simulink model "DR18E_Testpult"  (R2017a)
settings: Solver=ode1  StartTime=0.0  StopTime=Inf  FixedStep=0.001  RelTol=1e-3
PostLoadFcn:
  | , if any(exist('dsrtsu_mdlpostloadfcn', 'file') == [2, 3, 6]), try dsrtsu_mdlpostloadfcn('Execute', bdroot); catch fprintf('Error in PostLoadFcn (dsrtsu_mdlpostloadfcn) for model "%s":\n %s\n', bdroot, lasterr); end, end,
model workspace: external: MATLAB File C:\Users\DeltaRacing\Documents\dSPACE\MABX_DR18E\Model\DR18E_MABX_Parameter.m (data not in the file)
values from neighbouring files (symbols this model uses):
  am = 1/Ts    (= 1)    [DR18E_MABX_Parameter.m]
  bm = K/Ts    (= 0.05)    [DR18E_MABX_Parameter.m]
  cf = 41350    [DR18E_MABX_Parameter.m]
  cr = 41350    [DR18E_MABX_Parameter.m]
  Derating_HV_Battery_Kapa = 1    [DR18E_MABX_Parameter.m]
  Derating_Start_km = 16    [DR18E_MABX_Parameter.m]
  Drive_Mode = 0    [DR18E_MABX_Parameter.m]
  g = 1    [DR18E_MABX_Parameter.m]
  Gas_Modus = 2    [DR18E_MABX_Parameter.m]
  HV_Power_max = 80    [DR18E_MABX_Parameter.m]
  i_Getriebe = 3.3    [DR18E_MABX_Parameter.m]
  i_Lenkgetriebe = 4.32    [DR18E_MABX_Parameter.m]
  K_SET = 1    [DR18E_MABX_Parameter.m]
  Kapazitaet_HV_Battery_kWh = 6.6    [DR18E_MABX_Parameter.m]
  KW_T_Soll = 37    [DR18E_MABX_Parameter.m]
  lf = 1.2    [DR18E_MABX_Parameter.m]
  lr = 1.15    [DR18E_MABX_Parameter.m]
  m = 310    [DR18E_MABX_Parameter.m]
  M_max = 150    [DR18E_MABX_Parameter.m]
  Power_Limit_onoff = 0    [DR18E_MABX_Parameter.m]
  Reifenradius = 0.2351    [DR18E_MABX_Parameter.m]
  Strecke_Endu_km = 22    [DR18E_MABX_Parameter.m]
  TC_Decr_Gas = 0.00005    (= 5e-05)    [DR18E_MABX_Parameter.m]
  TC_Derivative = 0.4    [DR18E_MABX_Parameter.m]
  TC_Incr_Gas = 0.005    [DR18E_MABX_Parameter.m]
  TC_On = 0    [DR18E_MABX_Parameter.m]
  TC_Relay_Off = 0.065    [DR18E_MABX_Parameter.m]
  TC_Relay_On = 0.07    [DR18E_MABX_Parameter.m]
  TV_Mode = 2    [DR18E_MABX_Parameter.m]
  TV_On = 0    [DR18E_MABX_Parameter.m]
  TV_Override = 1    [DR18E_MABX_Parameter.m]
  y = 0.8    [DR18E_MABX_Parameter.m]
undefined symbols (not defined in the file or in its folder): D, DiscIntNeverNeededParam, I, K_OL, P
libraries: simulink x288, rtican x105, rtiusbflightreclib x40, rti1401lib_dio_type3 x10, simulink_extras x10, rti1401lib_adc_type4 x8, rti1401lib_II_base x7
(part 16 of 28)

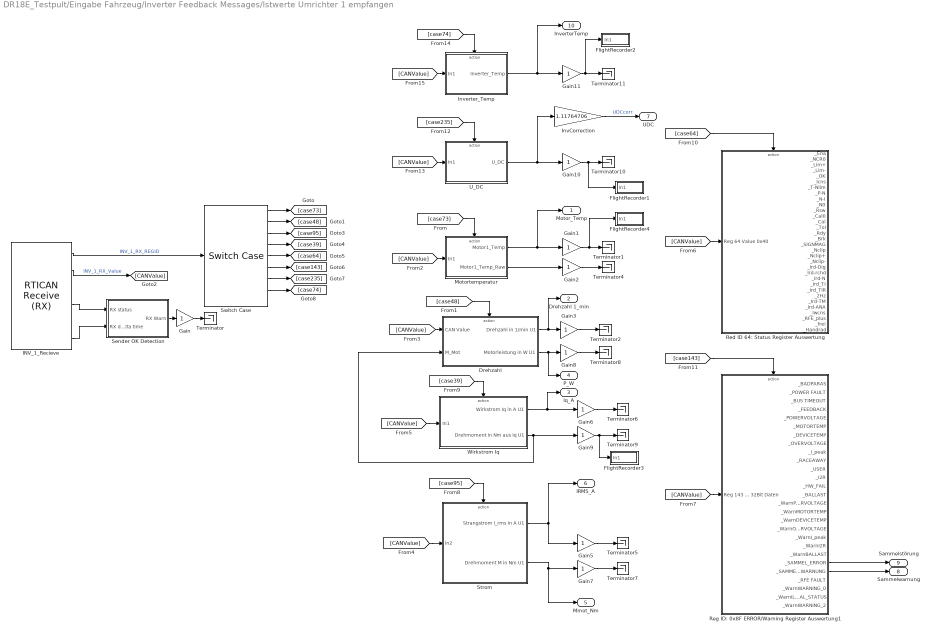
== system DR18E_Testpult/Eingabe Fahrzeug/Inverter Feedback Messages/Istwerte Umrichter 1 empfangen  ==
  Drehzahl : Subsystem  TreatAsAtomicUnit=on
  FlightRecorder1 : Subsystem
  FlightRecorder2 : Subsystem
  FlightRecorder3 : Subsystem
  FlightRecorder4 : Subsystem
  Gain{,1..3,5..11} (11 alike) : Gain
  INV_1_Recieve : rtican/RTICAN Receive (RX)   Reserved1=[]  Reserved2=[]  Reserved3=[]  Reserved4=[]  SfcnMessage=[]  Msg_Struct=[]  BoardTypeNo=[]  BoardNo=[]  ChannelNo=[]  Parameters=[]  DialogFcn=[]  UnitName=[]  Revision=[]  UnitValues=[]  DSProperties=struct('RTI',struct('Version',uint32(5),'BlockType',struct('isSLSource',uint8(1),'isSLSink',uint8(1),'isHWSource',uint8(0),'isHWSink',uint8(0),'isSetup',uint8(0),'isInline',uint8(1),'isNonInline',uint8(0),'isInterrupt',uint8(0),'isChannelwise',uint8(0)),'IOBoardType','RTICAN','UnitType','MESSAGE','Identifier','RX','DialogType','MSVC','BlockSet','RTICAN','SlaveProcessor','CAN'))  RTIBlockInterface=struct('OutputPortsWidth',int32([1 1 1 1 1 1]),'OutputPortsActive',[1 1 1 1 1 1],'OutputPortsName',{{'INV_1_RX_REGID','INV_1_RX_Value','muell',['RX status'],['RX time'],['RX delta time']}},'OutputPortsDataType',{{'SS_DOUBLE','SS_DOUBLE','SS_DOUBLE','SS_DOUBLE','SS_DOUBLE','SS_DOUBLE'}},'OutputPortsLabel',{{'INV_1_RX_REGID','INV_1_RX_Value','muell','','',''}},'OutputPortsLabelMode','ON','InputPortsWidth',int32(0),'InputPortsActive',0,'DialogFcn','rtican_message_interface_gui','BlockDisplay',{{'','center'}},'IconTransparency','on','ParameterTunableNames',{{}},'InitLevel',3,'BlockName',struct('Token',{{'INV_1_Recieve'}}),'SampleTime',{{-1}},'TriggerPort',{{'none'}},'EnablePort',{{'none'}})  RTIBlockParameters=struct('BoardTypeNo',{{1,'OFF',[]}},'BoardNo',{{1,'ON',[1 16]}},'ChannelNo',{{1,'ON',[1 2]}},'Parameters',{{struct('DataFileSupport',struct('DataFileSelectedMaster',0,'DataFileSelectedLocal',0,'DataFileName',['<no datafile support>|'],'DataFileDate',['01-Aug-2018 13:44:51'],'SelectedFile',['<no file selected>'],'InterfaceFcn','rtican_dbc_file_parser'),'Options',struct('StatusSelected',1,'TimeSelected',1,'DeltaTimeSelected',1,'BytePortSelected',0,'MessageLengthSelected',0,'TriggerPort',struct('Selected',0,'TriggerType',0),'UserCoding',struct('Selected',0,'InterfaceFile','UserDecodingFile','FcnName','UserDecodeFcn','InportSelected',0,'InportWidth',1,'OutportSelected',0,'OutportWidth',1),'EnablePortSelected',0,'SignalOnPortnameSelected',1,'UseRXService',0),'Message',struct('MsgOnBlocknameSelected',1,'MsgName','INV_1_Recieve','MsgIdFormat',0,'MsgId',273,'MsgLength',6,'NumSignals',3,'SampleTime',-1,'Signal',struct('SgnName',{'INV_1_RX_REGID','INV_1_RX_Value','muell'},'SgnStartBit',{0,8,40},'SgnLength',{8,16,8},'SgnType',{0,0,0},'ModeValue',{-1,-1,-1},'DataType',{0,0,0},'ByteLayout',{0,0,0},'Factor',{1,1,1},'Offset',{0,0,0},'SgnComment',{{''},{''},{''}},'SgnUnit',{'','',''},'Min',{0,0,0},'Max',{0,0,0},'SLDataType',{'SS_DOUBLE','SS_DOUBLE','SS_DOUBLE'}),'MsgIdNumFormat',1,'MsgComment',{{''}}),'Version',1.2,'general',struct('isFromLib',0)),'OFF',[]}},'GroupId',{{struct('Group',{{'RTICAN'}},'No',2,'Behavior',{{'NAMECHANGE'}},'BlockType',{{'SINK'}},'NameChangeFlag',0),'OFF',[]}},'SFcnRTICANMessage',{{struct('MsgType','RX','SFcnPortType','Scalar','MsgName','INV_1_Recieve','MsgIdFormat','STD','MsgId',273,'MsgLength',6,'NumSignals',3,'SampleTime',-1,'Signal',struct('SgnName',{'INV_1_RX_REGID','INV_1_RX_Value','muell'},'SgnStartBit',{0,8,40},'SgnLength',{8,16,8},'SgnType',{'standard','standard','standard'},'ModeValue',{-1,-1,-1},'DataType',{['unsigned int'],['unsigned int'],['unsigned int']},'ByteLayout',{['little endian'],['little endian'],['little endian']},'Factor',{1,1,1},'Offset',{0,0,0},'SLDataType',{'SS_DOUBLE','SS_DOUBLE','SS_DOUBLE'}),'StatusSelected','yes','TimeSelected','yes','DeltaTimeSelected','yes','BytePortSelected','no','MessageLengthSelected','no','TriggerPort',struct('Selected','no','TriggerType',0),'UserCoding',struct('Selected','no','InterfaceFile','UserDecodingFile','FcnName','UserDecodeFcn','InportSelected','no','InportWidth',1,'OutportSelected','no','OutportWidth',1),'EnablePortSelected','no','UseRXService','no','BoardType','DS1','BoardNo',1,'ControllerNo',1),'OFF',[]}},'TLCFileName',{{'rtican_rx_message','OFF',[]}})  RTISFcnParameters=struct('SFcnRTICANMessage','struct','TLCFileName','char')  RTIBlockParaDefault=struct('BoardTypeNo',4302,'BoardNo',1,'ChannelNo',1,'Parameters',struct('DataFileSupport',struct('DataFileSelectedMaster',0,'DataFileSelectedLocal',0,'DataFileName','','DataFileDate','','SelectedFile',['<no file selected>']),'Options',struct('StatusSelected',1,'TimeSelected',1,'DeltaTimeSelected',1,'BytePortSelected',0,'MessageLengthSelected',0,'TriggerPort',struct('Selected',0,'TriggerType','rising'),'UserCoding',struct('Selected',0,'InterfaceFile','UserDecodingFile','FcnName','UserDecodeFcn','InportSelected',0,'InportWidth',1,'OutportSelected',0,'OutportWidth',1),'EnablePortSelected',0,'SignalOnPortnameSelected',1,'UseRXService',0),'Message',struct('MsgOnBlocknameSelected',0,'MsgName',['RX Message'],'MsgIdFormat',0,'MsgId',100,'MsgLength',8,'NumSignals',1,'SampleTime',-1,'Signal',struct('SgnName',['RX signal'],'SgnStartBit',0,'SgnLength',8,'SgnType',0,'ModeValue',-1,'DataType',0,'SLDataType','SS_DOUBLE','ByteLayout',0,'Factor',1,'Offset',0,'Min',0,'Max',255,'SgnComment',{{}},'SgnUnit',''),'MsgIdNumFormat',0,'MsgComment',{{''}}),'Version',1.2,'general',struct('isFromLib',1)),'GroupId',struct('Group',{{'RTICAN'}},'No',1,'Behavior',{{'NAMECHANGE'}},'BlockType',{{'SINK'}},'NameChangeFlag',0),'SFcnRTICANMessage',struct('MsgType','RX','MsgName',['RX Message'],'MsgIdFormat','STD','MsgId',100,'MsgLength',8,'NumSignals',1,'SampleTime',-1,'Signal',struct('SgnName',['RX signal'],'SgnStartBit',0,'SgnLength',8,'SgnType','standard','ModeValue',-1,'DataType',['unsigned int'],'ByteLayout',['little endian'],'SLDataType','SS_DOUBLE','Factor',1,'Offset',0),'StatusSelected','yes','TimeSelected','yes','DeltaTimeSelected','yes','BytePortSelected','no','MessageLengthSelected','no','EnablePortSelected','no','UserCoding',struct('Selected','no','InterfaceFile','UserDecodingFile','FcnName','UserDecodeFcn','InportSelected','no','InportWidth',1,'OutportSelected','no','OutportWidth',1),'TriggerPort',struct('Selected','no','TriggerType','rising'),'UseRXService','no','BoardType','DS4302','BoardNo',1,'ControllerNo',1,'SFcnPortType','Scalar'),'TLCFileName','rtican_rx_message')
      settings: AttributesFormatString=Group Id: RTICAN2\n  SourceProductName=dSPACE RTI CAN Blockset
  InvCorrection : Gain  Gain=1.11764706
  Inverter_Temp : Subsystem  TreatAsAtomicUnit=on
  Motortemperatur : Subsystem  TreatAsAtomicUnit=on
  Red ID 64: Status Register Auswertung : Subsystem  TreatAsAtomicUnit=on
  Reg ID: 0x8F ERROR/Warning Register Auswertung1 : Subsystem  TreatAsAtomicUnit=on
  Sender OK Detection : Subsystem
  Strom : Subsystem  TreatAsAtomicUnit=on
  Switch Case : SwitchCase  CaseConditions={hex2dec('0049'),hex2dec('0030'),hex2dec('005F'),hex2dec('27'),64,hex2dec('8F'),hex2dec('EB'),hex2dec('4A')}
  Terminator{,1..2,4..11} (11 alike) : Terminator
  U_DC : Subsystem  TreatAsAtomicUnit=on
  Wirkstrom Iq : Subsystem  TreatAsAtomicUnit=on
  Motor_Temp : Outport
  Drehzahl 1_min : Outport  Port=2
  Iq_A : Outport  Port=3
  P_W : Outport  Port=4
  Mmot_Nm : Outport  Port=5
  IRMS_A : Outport  Port=6
  UDC : Outport  Port=7
  Sammelwarnung : Outport  Port=8
  Sammelstörung : Outport  Port=9
  InverterTemp : Outport  Port=10
  wires:
  Gain1/1 -> FlightRecorder4/1(In1), Terminator1/1
  Motortemperatur/2("Motor1_Temp_Raw ") -> Gain2/1
  Gain2/1 -> Terminator4/1
  Gain3/1 -> Terminator2/1
  Gain5/1 -> Terminator5/1
  Gain6/1 -> Terminator6/1
  Wirkstrom Iq/1(Wirkstrom Iq in A U1) -> Iq_A/1, Gain6/1
  Strom/1(Strangstrom I_rms in A U1) -> Gain5/1, IRMS_A/1
  Gain7/1 -> Terminator7/1
  Strom/2(Drehmoment M in Nm U1) -> Mmot_Nm/1, Gain7/1
  Gain8/1 -> Terminator8/1
  Drehzahl/1(Drehzahl in 1/min U1) -> Drehzahl 1_min/1, Gain3/1
  Drehzahl/2(Motorleistung in W U1) -> P_W/1, Gain8/1
  Sender OK Detection/1(RX Warn) -> Gain/1
  Gain/1 -> Terminator/1
  INV_1_Recieve/4 -> Sender OK Detection/1(RX status)
  INV_1_Recieve/6 -> Sender OK Detection/2(RX delta time)
  Gain9/1 -> FlightRecorder3/1(In1), Terminator9/1
  Wirkstrom Iq/2(Drehmoment in Nm aus Iq U1) -> Drehzahl/2(M_Mot), Gain9/1
  Switch Case/1 -> [case73]
  [case73] -> Motortemperatur/Action
  Switch Case/2 -> [case48]
  [case48] -> Drehzahl/Action
  [CANValue] -> Motortemperatur/1(In1)
  [CANValue] -> Drehzahl/1(CAN Value)
  [CANValue] -> Strom/1(In2)
  [CANValue] -> Wirkstrom Iq/1(In1)
  [CANValue] -> Red ID 64: Status Register Auswertung/1(Reg 64 Value 0x40)
  [CANValue] -> Reg ID: 0x8F ERROR/Warning Register Auswertung1/1(Reg 143 Value 0x8F 32Bit Daten)
  Switch Case/3 -> [case95]
  [case95] -> Strom/Action
  Switch Case/4 -> [case39]
  [case39] -> Wirkstrom Iq/Action
  [case64] -> Red ID 64: Status Register Auswertung/Action
  Switch Case/5 -> [case64]
  Switch Case/6 -> [case143]
  [case143] -> Reg ID: 0x8F ERROR/Warning Register Auswertung1/Action
  Motortemperatur/1(Motor1_Temp) -> Motor_Temp/1, Gain1/1
  Reg ID: 0x8F ERROR/Warning Register Auswertung1/23(_SAMMEL_WARNUNG) -> Sammelwarnung/1
  Reg ID: 0x8F ERROR/Warning Register Auswertung1/22(_SAMMEL_ERROR) -> Sammelstörung/1
  Switch Case/7 -> [case235]
  Gain10/1 -> FlightRecorder1/1(In1), Terminator10/1
  [case235] -> U_DC/Action
  [CANValue] -> U_DC/1(In1)
  U_DC/1(U_DC) -> InvCorrection/1, Gain10/1
  Switch Case/8 -> [case74]
  Gain11/1 -> FlightRecorder2/1(In1), Terminator11/1
  [case74] -> Inverter_Temp/Action
  [CANValue] -> Inverter_Temp/1(In1)
  Inverter_Temp/1(Inverter_Temp) -> InverterTemp/1, Gain11/1
  InvCorrection/1 -> UDC/1  "UDCcorr"
  INV_1_Recieve/2 -> [CANValue]  "INV_1_RX_Value"
  INV_1_Recieve/1 -> Switch Case/1  "INV_1_RX_REGID"

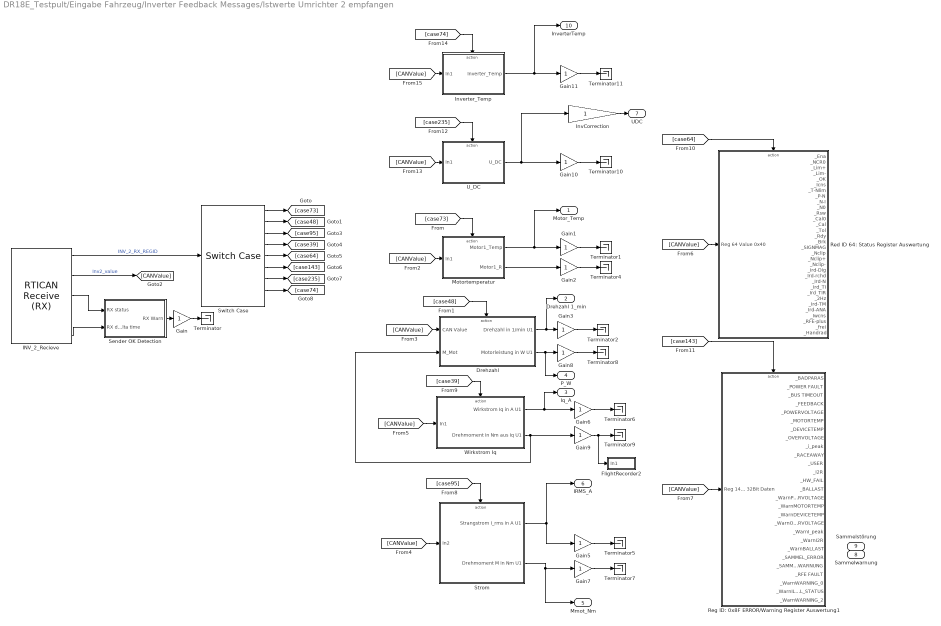
== system DR18E_Testpult/Eingabe Fahrzeug/Inverter Feedback Messages/Istwerte Umrichter 2 empfangen ==
  Drehzahl : Subsystem  TreatAsAtomicUnit=on
  FlightRecorder2 : Subsystem
  Gain{,1..3,5..11} (11 alike) : Gain
  INV_2_Recieve : rtican/RTICAN Receive (RX)   Reserved1=[]  Reserved2=[]  Reserved3=[]  Reserved4=[]  SfcnMessage=[]  Msg_Struct=[]  BoardTypeNo=[]  BoardNo=[]  ChannelNo=[]  Parameters=[]  DialogFcn=[]  UnitName=[]  Revision=[]  UnitValues=[]  DSProperties=struct('RTI',struct('Version',uint32(5),'BlockType',struct('isSLSource',uint8(1),'isSLSink',uint8(1),'isHWSource',uint8(0),'isHWSink',uint8(0),'isSetup',uint8(0),'isInline',uint8(1),'isNonInline',uint8(0),'isInterrupt',uint8(0),'isChannelwise',uint8(0)),'IOBoardType','RTICAN','UnitType','MESSAGE','Identifier','RX','DialogType','MSVC','BlockSet','RTICAN','SlaveProcessor','CAN'))  RTIBlockInterface=struct('OutputPortsWidth',int32([1 1 1 1 1]),'OutputPortsActive',[1 1 1 1 1],'OutputPortsName',{{'INV_2_RX_REGID','Inv2_value',['RX status'],['RX time'],['RX delta time']}},'OutputPortsDataType',{{'SS_DOUBLE','SS_DOUBLE','SS_DOUBLE','SS_DOUBLE','SS_DOUBLE'}},'OutputPortsLabel',{{'INV_2_RX_REGID','Inv2_value','','',''}},'OutputPortsLabelMode','ON','InputPortsWidth',int32(0),'InputPortsActive',0,'DialogFcn','rtican_message_interface_gui','BlockDisplay',{{'','center'}},'IconTransparency','on','ParameterTunableNames',{{}},'InitLevel',3,'BlockName',struct('Token',{{'INV_2_Recieve'}}),'SampleTime',{{-1}},'TriggerPort',{{'none'}},'EnablePort',{{'none'}})  RTIBlockParameters=struct('BoardTypeNo',{{1,'OFF',[]}},'BoardNo',{{1,'ON',[1 16]}},'ChannelNo',{{2,'ON',[1 2]}},'Parameters',{{struct('DataFileSupport',struct('DataFileSelectedMaster',0,'DataFileSelectedLocal',0,'DataFileName',['<no datafile support>|'],'DataFileDate',['01-Aug-2018 13:44:51'],'SelectedFile',['<no file selected>'],'InterfaceFcn','rtican_dbc_file_parser'),'Options',struct('StatusSelected',1,'TimeSelected',1,'DeltaTimeSelected',1,'BytePortSelected',0,'MessageLengthSelected',0,'TriggerPort',struct('Selected',0,'TriggerType',0),'UserCoding',struct('Selected',0,'InterfaceFile','UserDecodingFile','FcnName','UserDecodeFcn','InportSelected',0,'InportWidth',1,'OutportSelected',0,'OutportWidth',1),'EnablePortSelected',0,'SignalOnPortnameSelected',1,'UseRXService',0),'Message',struct('MsgOnBlocknameSelected',1,'MsgName','INV_2_Recieve','MsgIdFormat',0,'MsgId',274,'MsgLength',6,'NumSignals',2,'SampleTime',-1,'Signal',struct('SgnName',{'INV_2_RX_REGID','Inv2_value'},'SgnStartBit',{0,8},'SgnLength',{8,16},'SgnType',{0,0},'ModeValue',{-1,-1},'DataType',{0,0},'ByteLayout',{0,0},'Factor',{1,1},'Offset',{0,0},'SgnComment',{{''},{''}},'SgnUnit',{'',''},'Min',{0,0},'Max',{0,0},'SLDataType',{'SS_DOUBLE','SS_DOUBLE'}),'MsgIdNumFormat',1,'MsgComment',{{''}}),'Version',1.2,'general',struct('isFromLib',0)),'OFF',[]}},'GroupId',{{struct('Group',{{'RTICAN'}},'No',3,'Behavior',{{'NAMECHANGE'}},'BlockType',{{'SINK'}},'NameChangeFlag',0),'OFF',[]}},'SFcnRTICANMessage',{{struct('MsgType','RX','SFcnPortType','Scalar','MsgName','INV_2_Recieve','MsgIdFormat','STD','MsgId',274,'MsgLength',6,'NumSignals',2,'SampleTime',-1,'Signal',struct('SgnName',{'INV_2_RX_REGID','Inv2_value'},'SgnStartBit',{0,8},'SgnLength',{8,16},'SgnType',{'standard','standard'},'ModeValue',{-1,-1},'DataType',{['unsigned int'],['unsigned int']},'ByteLayout',{['little endian'],['little endian']},'Factor',{1,1},'Offset',{0,0},'SLDataType',{'SS_DOUBLE','SS_DOUBLE'}),'StatusSelected','yes','TimeSelected','yes','DeltaTimeSelected','yes','BytePortSelected','no','MessageLengthSelected','no','TriggerPort',struct('Selected','no','TriggerType',0),'UserCoding',struct('Selected','no','InterfaceFile','UserDecodingFile','FcnName','UserDecodeFcn','InportSelected','no','InportWidth',1,'OutportSelected','no','OutportWidth',1),'EnablePortSelected','no','UseRXService','no','BoardType','DS1','BoardNo',1,'ControllerNo',2),'OFF',[]}},'TLCFileName',{{'rtican_rx_message','OFF',[]}})  RTISFcnParameters=struct('SFcnRTICANMessage','struct','TLCFileName','char')  RTIBlockParaDefault=struct('BoardTypeNo',4302,'BoardNo',1,'ChannelNo',1,'Parameters',struct('DataFileSupport',struct('DataFileSelectedMaster',0,'DataFileSelectedLocal',0,'DataFileName','','DataFileDate','','SelectedFile',['<no file selected>']),'Options',struct('StatusSelected',1,'TimeSelected',1,'DeltaTimeSelected',1,'BytePortSelected',0,'MessageLengthSelected',0,'TriggerPort',struct('Selected',0,'TriggerType','rising'),'UserCoding',struct('Selected',0,'InterfaceFile','UserDecodingFile','FcnName','UserDecodeFcn','InportSelected',0,'InportWidth',1,'OutportSelected',0,'OutportWidth',1),'EnablePortSelected',0,'SignalOnPortnameSelected',1,'UseRXService',0),'Message',struct('MsgOnBlocknameSelected',0,'MsgName',['RX Message'],'MsgIdFormat',0,'MsgId',100,'MsgLength',8,'NumSignals',1,'SampleTime',-1,'Signal',struct('SgnName',['RX signal'],'SgnStartBit',0,'SgnLength',8,'SgnType',0,'ModeValue',-1,'DataType',0,'SLDataType','SS_DOUBLE','ByteLayout',0,'Factor',1,'Offset',0,'Min',0,'Max',255,'SgnComment',{{}},'SgnUnit',''),'MsgIdNumFormat',0,'MsgComment',{{''}}),'Version',1.2,'general',struct('isFromLib',1)),'GroupId',struct('Group',{{'RTICAN'}},'No',1,'Behavior',{{'NAMECHANGE'}},'BlockType',{{'SINK'}},'NameChangeFlag',0),'SFcnRTICANMessage',struct('MsgType','RX','MsgName',['RX Message'],'MsgIdFormat','STD','MsgId',100,'MsgLength',8,'NumSignals',1,'SampleTime',-1,'Signal',struct('SgnName',['RX signal'],'SgnStartBit',0,'SgnLength',8,'SgnType','standard','ModeValue',-1,'DataType',['unsigned int'],'ByteLayout',['little endian'],'SLDataType','SS_DOUBLE','Factor',1,'Offset',0),'StatusSelected','yes','TimeSelected','yes','DeltaTimeSelected','yes','BytePortSelected','no','MessageLengthSelected','no','EnablePortSelected','no','UserCoding',struct('Selected','no','InterfaceFile','UserDecodingFile','FcnName','UserDecodeFcn','InportSelected','no','InportWidth',1,'OutportSelected','no','OutportWidth',1),'TriggerPort',struct('Selected','no','TriggerType','rising'),'UseRXService','no','BoardType','DS4302','BoardNo',1,'ControllerNo',1,'SFcnPortType','Scalar'),'TLCFileName','rtican_rx_message')
      settings: AttributesFormatString=Group Id: RTICAN3\n  SourceProductName=dSPACE RTI CAN Blockset
  InvCorrection : Gain
  Inverter_Temp : Subsystem  TreatAsAtomicUnit=on
  Motortemperatur : Subsystem  TreatAsAtomicUnit=on
  Red ID 64: Status Register Auswertung : Subsystem  TreatAsAtomicUnit=on
  Reg ID: 0x8F ERROR/Warning Register Auswertung1 : Subsystem  TreatAsAtomicUnit=on
  Sender OK Detection : Subsystem
  Strom : Subsystem  TreatAsAtomicUnit=on
  Switch Case : SwitchCase  CaseConditions={hex2dec('0049'),hex2dec('0030'),hex2dec('005F'),hex2dec('27'),64,hex2dec('8F'),hex2dec('EB'),hex2dec('4A')}
  Terminator{,1..2,4..11} (11 alike) : Terminator
  U_DC : Subsystem  TreatAsAtomicUnit=on
  Wirkstrom Iq : Subsystem  TreatAsAtomicUnit=on
  Motor_Temp : Outport
  Drehzahl 1_min : Outport  Port=2
  Iq_A : Outport  Port=3
  P_W : Outport  Port=4
  Mmot_Nm : Outport  Port=5
  IRMS_A : Outport  Port=6
  UDC : Outport  Port=7
  Sammelwarnung : Outport  Port=8
  Sammelstörung : Outport  Port=9
  InverterTemp : Outport  Port=10
  wires:
  Gain1/1 -> Terminator1/1
  Motortemperatur/2("Motor1_R ") -> Gain2/1
  Gain2/1 -> Terminator4/1
  Gain3/1 -> Terminator2/1
  Gain5/1 -> Terminator5/1
  Gain6/1 -> Terminator6/1
  Wirkstrom Iq/1(Wirkstrom Iq in A U1) -> Iq_A/1, Gain6/1
  Strom/1(Strangstrom I_rms in A U1) -> Gain5/1, IRMS_A/1
  Gain7/1 -> Terminator7/1
  Strom/2(Drehmoment M in Nm U1) -> Mmot_Nm/1, Gain7/1
  Gain8/1 -> Terminator8/1
  Drehzahl/1(Drehzahl in 1/min U1) -> Drehzahl 1_min/1, Gain3/1
  Drehzahl/2(Motorleistung in W U1) -> P_W/1, Gain8/1
  Sender OK Detection/1(RX Warn) -> Gain/1
  Gain/1 -> Terminator/1
  INV_2_Recieve/3 -> Sender OK Detection/1(RX status)
  INV_2_Recieve/5 -> Sender OK Detection/2(RX delta time)
  Gain9/1 -> FlightRecorder2/1(In1), Terminator9/1
  Wirkstrom Iq/2(Drehmoment in Nm aus Iq U1) -> Drehzahl/2(M_Mot), Gain9/1
  Switch Case/1 -> [case73]
  [case73] -> Motortemperatur/Action
  Switch Case/2 -> [case48]
  [case48] -> Drehzahl/Action
  [CANValue] -> Motortemperatur/1(In1)
  [CANValue] -> Drehzahl/1(CAN Value)
  [CANValue] -> Strom/1(In2)
  [CANValue] -> Wirkstrom Iq/1(In1)
  [CANValue] -> Red ID 64: Status Register Auswertung/1(Reg 64 Value 0x40)
  [CANValue] -> Reg ID: 0x8F ERROR/Warning Register Auswertung1/1(Reg 143 Value 0x8F 32Bit Daten)
  Switch Case/3 -> [case95]
  [case95] -> Strom/Action
  Switch Case/4 -> [case39]
  [case39] -> Wirkstrom Iq/Action
  [case64] -> Red ID 64: Status Register Auswertung/Action
  Switch Case/5 -> [case64]
  Switch Case/6 -> [case143]
  [case143] -> Reg ID: 0x8F ERROR/Warning Register Auswertung1/Action
  Motortemperatur/1(Motor1_Temp) -> Motor_Temp/1, Gain1/1
  ? -> Sammelwarnung/1
  ? -> Sammelstörung/1
  Switch Case/7 -> [case235]
  Gain10/1 -> Terminator10/1
  [case235] -> U_DC/Action
  [CANValue] -> U_DC/1(In1)
  U_DC/1(U_DC) -> InvCorrection/1, Gain10/1
  Switch Case/8 -> [case74]
  Gain11/1 -> Terminator11/1
  [case74] -> Inverter_Temp/Action
  [CANValue] -> Inverter_Temp/1(In1)
  Inverter_Temp/1(Inverter_Temp) -> InverterTemp/1, Gain11/1
  InvCorrection/1 -> UDC/1
  INV_2_Recieve/1 -> Switch Case/1  "INV_2_RX_REGID"
  INV_2_Recieve/2 -> [CANValue]  "Inv2_value"

== system DR18E_Testpult/Eingabe Fahrzeug/Lenkwinkelgeber/FlightRecorder ==
  In1 : Inport
  Data Type Conversion : DataTypeConversion
  Gain : Gain
  USB_FLIGHT_REC_BL1 : rtiusbflightreclib/USB_FLIGHT_REC_BL1  VarName=Lenkwinkel  DataType=Single  SampleTime=-1  TLCFileName=rtiusbflightrecwrite  Reserved1=[]  Reserved2=[]  Reserved3=[]  Reserved4=[]  DSProperties=struct('RTI',struct('Version',uint32(3),'BlockType',struct('isSLSource',uint8(0),'isSLSink',uint8(1),'isHWSource',uint8(0),'isHWSink',uint8(0),'isSetup',uint8(0),'isInline',uint8(1),'isNonInline',uint8(0),'isInterrupt',uint8(0),'isChannelwise',uint8(0)),'IOBoardType',{{'DSUSB','FLIGHTREC'}},'UnitType','FLIGHTREC','Identifier','WRITE','DialogType','SL','BlockSet','RTIUSBFLIGHTREC','SlaveProcessor','NONE'))  RTIBlockInterface=struct('InputPortsActive',1,'InputPortsWidth',int32(1),'InputPortsDataType',{{'SS_SINGLE'}},'BlockDisplay',{{['Write to\nUSB Flight Recorder'],'center'}},'IconTransparency','off','InitLevel',3,'BlockName',struct('Token',{{'USB_FLIGHT_REC_BL1'}}),'MaskDescription',['Write input to the Flight Recorder. Recorded data can be referenced by the specified variable.'],'SampleTime',{{-1}})  RTIBlockParameters=struct('VarName',{{'Lenkwinkel','OFF',[]}},'DataType',{{'Single','OFF',[]}},'SampleTime',{{-1,'OFF',[]}},'TLCFileName',{{'rtiusbflightrecwrite','OFF',[]}})  RTISFcnParameters=struct('VarName','char','DataType','char','SampleTime','double','TLCFileName','char')  RTIBlockParaDefault=struct('VarName','Var1','DataType','Single','SampleTime',-1,'TLCFileName','rtiusbflightrecwrite')
      settings: SourceProductName=dSPACE RTI USB Flight Rec Blockset
  wires:
  Data Type Conversion/1 -> USB_FLIGHT_REC_BL1/1
  In1/1 -> Gain/1
  Gain/1 -> Data Type Conversion/1

== system DR18E_Testpult/Eingabe Fahrzeug/Lenkwinkelgeber/RX Timeout Detection ==
  RX status : Inport
  Timeout (n Samples) : Inport  Port=2
  Terminator_4 : Terminator
  Triggered Subsystem : Subsystem  TreatAsAtomicUnit=on
  RX Timeout Error : Outport
  wires:
  RX status/1 -> Triggered Subsystem/1(TXStatus)
  Triggered Subsystem/1(Rampe) -> Terminator_4/1
  Triggered Subsystem/2(RX Timeout Error) -> RX Timeout Error/1  "RX Timeout"
  Timeout (n Samples)/1 -> Triggered Subsystem/2(Timeout)

== system DR18E_Testpult/Eingabe Fahrzeug/MicroAutoBox/AI ==
  ADC_TYPE4_BL1 : rti1401lib_adc_type4/ADC_TYPE4_BL1  DSProperties=struct('RTI',struct('Version',uint32(2),'BlockType',struct('isSLSource',uint8(1),'isSLSink',uint8(1),'isHWSource',uint8(0),'isHWSink',uint8(1),'isSetup',uint8(0),'isInline',uint8(1),'isNonInline',uint8(0),'isInterrupt',uint8(0),'isChannelwise',uint8(1)),'IOBoardType',{{'DS1401','STD','ADCT4'}},'UnitType','ADC','Identifier','ADC','DialogType','ML','BlockSet','NONE','SlaveProcessor','NONE'))  RTIBlockInterface=struct('InputPortsActive',0,'InputPortsWidth',int32(1),'InputPortsDataType',{{'SS_BOOLEAN'}},'InputPortsName',{{'Continue'}},'OutputPortsActive',[1 0],'OutputPortsWidth',int32([1 1]),'OutputPortsDataType',{{'SS_DOUBLE','SS_UINT8'}},'OutputPortsName',{{'ADC','Status'}},'DialogFcn','rti1401stdadct4adcgui','SampleTime',{{0.1}},'InitLevel',3,'IconTransparency','on','BlockDisplay',{{['ADC TP4\nModule: 1\nChannel: 1'],'center'}},'BlockName',struct('Token',{{'ADC_TYPE4_BL1'}}))  RTIBlockParameters=struct('ADCSWStartDisable',{{0,'OFF',[0 1]}},'ModuleNo',{{1,'OFF',[1 16]}},'ChannelNo',{{1,'OFF',[1 16]}},'ConversionMode',{{1,'OFF',[1 2]}},'SampleMode',{{1,'OFF',[1 2]}},'TriggerSource',{{1,'OFF',[1 5]}},'EdgePolarity',{{1,'OFF',[1 2]}},'ConversionTriggerSource',{{2,'OFF',[1 6]}},'ConversionEdgePolarity',{{1,'OFF',[1 2]}},'ConversionPeriod',{{'1e-06','OFF',[]}},'ConversionPeriodCheck',{{0,'OFF',[]}},'BurstTriggerSource',{{1,'OFF',[1 6]}},'BurstEdgePolarity',{{1,'OFF',[1 2]}},'BurstSize',{{'10','OFF',[]}},'BurstSizeCheck',{{0,'OFF',[]}},'DataSetOffset',{{'0','OFF',[]}},'DataSetOffsetCheck',{{0,'OFF',[]}},'DataSetLength',{{'1','OFF',[]}},'DataSetLengthCheck',{{0,'OFF',[]}},'ReadMode',{{1,'OFF',[1 2]}},'SampleTime',{{'100e-3','OFF',[-1 inf]}},'SampleTimeCheck',{{1,'OFF',[]}},'StatusPortEnable',{{0,'OFF',[0 1]}},'TLCFileName',{{'rti1401adc_t4_adc','OFF',[]}},'VoltageRange',{{1,'OFF',[1 2]}})  RTISFcnParameters=struct('ADCSWStartDisable','int32','ModuleNo','int32','ChannelNo','int16','ConversionMode','int16','SampleMode','int16','TriggerSource','int16','EdgePolarity','int16','ConversionTriggerSource','int16','ConversionEdgePolarity','int16','ConversionPeriod','double','BurstTriggerSource','int16','BurstEdgePolarity','int16','BurstSize','int16','DataSetOffset','int16','DataSetLength','int16','ReadMode','int16','SampleTime','double','StatusPortEnable','int16','TLCFileName','char','VoltageRange','int16')  RTIBlockParaDefault=struct('ADCSWStartDisable',0,'ModuleNo',1,'ChannelNo',1,'ConversionMode',1,'SampleMode',1,'TriggerSource',1,'EdgePolarity',1,'ConversionTriggerSource',2,'ConversionEdgePolarity',1,'ConversionPeriod',1e-6,'ConversionPeriodCheck',0,'BurstTriggerSource',1,'BurstEdgePolarity',1,'BurstSize',10,'BurstSizeCheck',0,'DataSetOffset',0,'DataSetOffsetCheck',0,'DataSetLength',1,'DataSetLengthCheck',0,'ReadMode',1,'SampleTime',-1,'SampleTimeCheck',1,'StatusPortEnable',0,'TLCFileName','rti1401adc_t4_adc','VoltageRange',1)
  ADC_TYPE4_BL2 : rti1401lib_adc_type4/ADC_TYPE4_BL1  DSProperties=struct('RTI',struct('Version',uint32(2),'BlockType',struct('isSLSource',uint8(1),'isSLSink',uint8(1),'isHWSource',uint8(0),'isHWSink',uint8(1),'isSetup',uint8(0),'isInline',uint8(1),'isNonInline',uint8(0),'isInterrupt',uint8(0),'isChannelwise',uint8(1)),'IOBoardType',{{'DS1401','STD','ADCT4'}},'UnitType','ADC','Identifier','ADC','DialogType','ML','BlockSet','NONE','SlaveProcessor','NONE'))  RTIBlockInterface=struct('InputPortsActive',0,'InputPortsWidth',int32(1),'InputPortsDataType',{{'SS_BOOLEAN'}},'InputPortsName',{{'Continue'}},'OutputPortsActive',[1 0],'OutputPortsWidth',int32([1 1]),'OutputPortsDataType',{{'SS_DOUBLE','SS_UINT8'}},'OutputPortsName',{{'ADC','Status'}},'DialogFcn','rti1401stdadct4adcgui','SampleTime',{{0.1}},'InitLevel',3,'IconTransparency','on','BlockDisplay',{{['ADC TP4\nModule: 1\nChannel: 2'],'center'}},'BlockName',struct('Token',{{'ADC_TYPE4_BL1'}}))  RTIBlockParameters=struct('ADCSWStartDisable',{{0,'OFF',[0 1]}},'ModuleNo',{{1,'OFF',[1 16]}},'ChannelNo',{{2,'OFF',[1 16]}},'ConversionMode',{{1,'OFF',[1 2]}},'SampleMode',{{1,'OFF',[1 2]}},'TriggerSource',{{1,'OFF',[1 5]}},'EdgePolarity',{{1,'OFF',[1 2]}},'ConversionTriggerSource',{{2,'OFF',[1 6]}},'ConversionEdgePolarity',{{1,'OFF',[1 2]}},'ConversionPeriod',{{'1e-06','OFF',[]}},'ConversionPeriodCheck',{{0,'OFF',[]}},'BurstTriggerSource',{{1,'OFF',[1 6]}},'BurstEdgePolarity',{{1,'OFF',[1 2]}},'BurstSize',{{'10','OFF',[]}},'BurstSizeCheck',{{0,'OFF',[]}},'DataSetOffset',{{'0','OFF',[]}},'DataSetOffsetCheck',{{0,'OFF',[]}},'DataSetLength',{{'1','OFF',[]}},'DataSetLengthCheck',{{0,'OFF',[]}},'ReadMode',{{1,'OFF',[1 2]}},'SampleTime',{{'100e-3','OFF',[-1 inf]}},'SampleTimeCheck',{{1,'OFF',[]}},'StatusPortEnable',{{0,'OFF',[0 1]}},'TLCFileName',{{'rti1401adc_t4_adc','OFF',[]}},'VoltageRange',{{1,'OFF',[1 2]}})  RTISFcnParameters=struct('ADCSWStartDisable','int32','ModuleNo','int32','ChannelNo','int16','ConversionMode','int16','SampleMode','int16','TriggerSource','int16','EdgePolarity','int16','ConversionTriggerSource','int16','ConversionEdgePolarity','int16','ConversionPeriod','double','BurstTriggerSource','int16','BurstEdgePolarity','int16','BurstSize','int16','DataSetOffset','int16','DataSetLength','int16','ReadMode','int16','SampleTime','double','StatusPortEnable','int16','TLCFileName','char','VoltageRange','int16')  RTIBlockParaDefault=struct('ADCSWStartDisable',0,'ModuleNo',1,'ChannelNo',1,'ConversionMode',1,'SampleMode',1,'TriggerSource',1,'EdgePolarity',1,'ConversionTriggerSource',2,'ConversionEdgePolarity',1,'ConversionPeriod',1e-6,'ConversionPeriodCheck',0,'BurstTriggerSource',1,'BurstEdgePolarity',1,'BurstSize',10,'BurstSizeCheck',0,'DataSetOffset',0,'DataSetOffsetCheck',0,'DataSetLength',1,'DataSetLengthCheck',0,'ReadMode',1,'SampleTime',-1,'SampleTimeCheck',1,'StatusPortEnable',0,'TLCFileName','rti1401adc_t4_adc','VoltageRange',1)
  ADC_TYPE4_BL3 : rti1401lib_adc_type4/ADC_TYPE4_BL1  DSProperties=struct('RTI',struct('Version',uint32(2),'BlockType',struct('isSLSource',uint8(1),'isSLSink',uint8(1),'isHWSource',uint8(0),'isHWSink',uint8(1),'isSetup',uint8(0),'isInline',uint8(1),'isNonInline',uint8(0),'isInterrupt',uint8(0),'isChannelwise',uint8(1)),'IOBoardType',{{'DS1401','STD','ADCT4'}},'UnitType','ADC','Identifier','ADC','DialogType','ML','BlockSet','NONE','SlaveProcessor','NONE'))  RTIBlockInterface=struct('InputPortsActive',0,'InputPortsWidth',int32(1),'InputPortsDataType',{{'SS_BOOLEAN'}},'InputPortsName',{{'Continue'}},'OutputPortsActive',[1 0],'OutputPortsWidth',int32([1 1]),'OutputPortsDataType',{{'SS_DOUBLE','SS_UINT8'}},'OutputPortsName',{{'ADC','Status'}},'DialogFcn','rti1401stdadct4adcgui','SampleTime',{{0.1}},'InitLevel',3,'IconTransparency','on','BlockDisplay',{{['ADC TP4\nModule: 1\nChannel: 3'],'center'}},'BlockName',struct('Token',{{'ADC_TYPE4_BL1'}}))  RTIBlockParameters=struct('ADCSWStartDisable',{{0,'OFF',[0 1]}},'ModuleNo',{{1,'OFF',[1 16]}},'ChannelNo',{{3,'OFF',[1 16]}},'ConversionMode',{{1,'OFF',[1 2]}},'SampleMode',{{1,'OFF',[1 2]}},'TriggerSource',{{1,'OFF',[1 5]}},'EdgePolarity',{{1,'OFF',[1 2]}},'ConversionTriggerSource',{{2,'OFF',[1 6]}},'ConversionEdgePolarity',{{1,'OFF',[1 2]}},'ConversionPeriod',{{'1e-06','OFF',[]}},'ConversionPeriodCheck',{{0,'OFF',[]}},'BurstTriggerSource',{{1,'OFF',[1 6]}},'BurstEdgePolarity',{{1,'OFF',[1 2]}},'BurstSize',{{'10','OFF',[]}},'BurstSizeCheck',{{0,'OFF',[]}},'DataSetOffset',{{'0','OFF',[]}},'DataSetOffsetCheck',{{0,'OFF',[]}},'DataSetLength',{{'1','OFF',[]}},'DataSetLengthCheck',{{0,'OFF',[]}},'ReadMode',{{1,'OFF',[1 2]}},'SampleTime',{{'100e-3','OFF',[-1 inf]}},'SampleTimeCheck',{{1,'OFF',[]}},'StatusPortEnable',{{0,'OFF',[0 1]}},'TLCFileName',{{'rti1401adc_t4_adc','OFF',[]}},'VoltageRange',{{1,'OFF',[1 2]}})  RTISFcnParameters=struct('ADCSWStartDisable','int32','ModuleNo','int32','ChannelNo','int16','ConversionMode','int16','SampleMode','int16','TriggerSource','int16','EdgePolarity','int16','ConversionTriggerSource','int16','ConversionEdgePolarity','int16','ConversionPeriod','double','BurstTriggerSource','int16','BurstEdgePolarity','int16','BurstSize','int16','DataSetOffset','int16','DataSetLength','int16','ReadMode','int16','SampleTime','double','StatusPortEnable','int16','TLCFileName','char','VoltageRange','int16')  RTIBlockParaDefault=struct('ADCSWStartDisable',0,'ModuleNo',1,'ChannelNo',1,'ConversionMode',1,'SampleMode',1,'TriggerSource',1,'EdgePolarity',1,'ConversionTriggerSource',2,'ConversionEdgePolarity',1,'ConversionPeriod',1e-6,'ConversionPeriodCheck',0,'BurstTriggerSource',1,'BurstEdgePolarity',1,'BurstSize',10,'BurstSizeCheck',0,'DataSetOffset',0,'DataSetOffsetCheck',0,'DataSetLength',1,'DataSetLengthCheck',0,'ReadMode',1,'SampleTime',-1,'SampleTimeCheck',1,'StatusPortEnable',0,'TLCFileName','rti1401adc_t4_adc','VoltageRange',1)
  ADC_TYPE4_BL4 : rti1401lib_adc_type4/ADC_TYPE4_BL1  DSProperties=struct('RTI',struct('Version',uint32(2),'BlockType',struct('isSLSource',uint8(1),'isSLSink',uint8(1),'isHWSource',uint8(0),'isHWSink',uint8(1),'isSetup',uint8(0),'isInline',uint8(1),'isNonInline',uint8(0),'isInterrupt',uint8(0),'isChannelwise',uint8(1)),'IOBoardType',{{'DS1401','STD','ADCT4'}},'UnitType','ADC','Identifier','ADC','DialogType','ML','BlockSet','NONE','SlaveProcessor','NONE'))  RTIBlockInterface=struct('InputPortsActive',0,'InputPortsWidth',int32(1),'InputPortsDataType',{{'SS_BOOLEAN'}},'InputPortsName',{{'Continue'}},'OutputPortsActive',[1 0],'OutputPortsWidth',int32([1 1]),'OutputPortsDataType',{{'SS_DOUBLE','SS_UINT8'}},'OutputPortsName',{{'ADC','Status'}},'DialogFcn','rti1401stdadct4adcgui','SampleTime',{{0.1}},'InitLevel',3,'IconTransparency','on','BlockDisplay',{{['ADC TP4\nModule: 1\nChannel: 4'],'center'}},'BlockName',struct('Token',{{'ADC_TYPE4_BL1'}}))  RTIBlockParameters=struct('ADCSWStartDisable',{{0,'OFF',[0 1]}},'ModuleNo',{{1,'OFF',[1 16]}},'ChannelNo',{{4,'OFF',[1 16]}},'ConversionMode',{{1,'OFF',[1 2]}},'SampleMode',{{1,'OFF',[1 2]}},'TriggerSource',{{1,'OFF',[1 5]}},'EdgePolarity',{{1,'OFF',[1 2]}},'ConversionTriggerSource',{{2,'OFF',[1 6]}},'ConversionEdgePolarity',{{1,'OFF',[1 2]}},'ConversionPeriod',{{'1e-06','OFF',[]}},'ConversionPeriodCheck',{{0,'OFF',[]}},'BurstTriggerSource',{{1,'OFF',[1 6]}},'BurstEdgePolarity',{{1,'OFF',[1 2]}},'BurstSize',{{'10','OFF',[]}},'BurstSizeCheck',{{0,'OFF',[]}},'DataSetOffset',{{'0','OFF',[]}},'DataSetOffsetCheck',{{0,'OFF',[]}},'DataSetLength',{{'1','OFF',[]}},'DataSetLengthCheck',{{0,'OFF',[]}},'ReadMode',{{1,'OFF',[1 2]}},'SampleTime',{{'100e-3','OFF',[-1 inf]}},'SampleTimeCheck',{{1,'OFF',[]}},'StatusPortEnable',{{0,'OFF',[0 1]}},'TLCFileName',{{'rti1401adc_t4_adc','OFF',[]}},'VoltageRange',{{1,'OFF',[1 2]}})  RTISFcnParameters=struct('ADCSWStartDisable','int32','ModuleNo','int32','ChannelNo','int16','ConversionMode','int16','SampleMode','int16','TriggerSource','int16','EdgePolarity','int16','ConversionTriggerSource','int16','ConversionEdgePolarity','int16','ConversionPeriod','double','BurstTriggerSource','int16','BurstEdgePolarity','int16','BurstSize','int16','DataSetOffset','int16','DataSetLength','int16','ReadMode','int16','SampleTime','double','StatusPortEnable','int16','TLCFileName','char','VoltageRange','int16')  RTIBlockParaDefault=struct('ADCSWStartDisable',0,'ModuleNo',1,'ChannelNo',1,'ConversionMode',1,'SampleMode',1,'TriggerSource',1,'EdgePolarity',1,'ConversionTriggerSource',2,'ConversionEdgePolarity',1,'ConversionPeriod',1e-6,'ConversionPeriodCheck',0,'BurstTriggerSource',1,'BurstEdgePolarity',1,'BurstSize',10,'BurstSizeCheck',0,'DataSetOffset',0,'DataSetOffsetCheck',0,'DataSetLength',1,'DataSetLengthCheck',0,'ReadMode',1,'SampleTime',-1,'SampleTimeCheck',1,'StatusPortEnable',0,'TLCFileName','rti1401adc_t4_adc','VoltageRange',1)
  ADC_TYPE4_BL5 : rti1401lib_adc_type4/ADC_TYPE4_BL1  DSProperties=struct('RTI',struct('Version',uint32(2),'BlockType',struct('isSLSource',uint8(1),'isSLSink',uint8(1),'isHWSource',uint8(0),'isHWSink',uint8(1),'isSetup',uint8(0),'isInline',uint8(1),'isNonInline',uint8(0),'isInterrupt',uint8(0),'isChannelwise',uint8(1)),'IOBoardType',{{'DS1401','STD','ADCT4'}},'UnitType','ADC','Identifier','ADC','DialogType','ML','BlockSet','NONE','SlaveProcessor','NONE'))  RTIBlockInterface=struct('InputPortsActive',0,'InputPortsWidth',int32(1),'InputPortsDataType',{{'SS_BOOLEAN'}},'InputPortsName',{{'Continue'}},'OutputPortsActive',[1 0],'OutputPortsWidth',int32([1 1]),'OutputPortsDataType',{{'SS_DOUBLE','SS_UINT8'}},'OutputPortsName',{{'ADC','Status'}},'DialogFcn','rti1401stdadct4adcgui','SampleTime',{{0.1}},'InitLevel',3,'IconTransparency','on','BlockDisplay',{{['ADC TP4\nModule: 1\nChannel: 5'],'center'}},'BlockName',struct('Token',{{'ADC_TYPE4_BL1'}}))  RTIBlockParameters=struct('ADCSWStartDisable',{{0,'OFF',[0 1]}},'ModuleNo',{{1,'OFF',[1 16]}},'ChannelNo',{{5,'OFF',[1 16]}},'ConversionMode',{{1,'OFF',[1 2]}},'SampleMode',{{1,'OFF',[1 2]}},'TriggerSource',{{1,'OFF',[1 5]}},'EdgePolarity',{{1,'OFF',[1 2]}},'ConversionTriggerSource',{{2,'OFF',[1 6]}},'ConversionEdgePolarity',{{1,'OFF',[1 2]}},'ConversionPeriod',{{'1e-06','OFF',[]}},'ConversionPeriodCheck',{{0,'OFF',[]}},'BurstTriggerSource',{{1,'OFF',[1 6]}},'BurstEdgePolarity',{{1,'OFF',[1 2]}},'BurstSize',{{'10','OFF',[]}},'BurstSizeCheck',{{0,'OFF',[]}},'DataSetOffset',{{'0','OFF',[]}},'DataSetOffsetCheck',{{0,'OFF',[]}},'DataSetLength',{{'1','OFF',[]}},'DataSetLengthCheck',{{0,'OFF',[]}},'ReadMode',{{1,'OFF',[1 2]}},'SampleTime',{{'100e-3','OFF',[-1 inf]}},'SampleTimeCheck',{{1,'OFF',[]}},'StatusPortEnable',{{0,'OFF',[0 1]}},'TLCFileName',{{'rti1401adc_t4_adc','OFF',[]}},'VoltageRange',{{1,'OFF',[1 2]}})  RTISFcnParameters=struct('ADCSWStartDisable','int32','ModuleNo','int32','ChannelNo','int16','ConversionMode','int16','SampleMode','int16','TriggerSource','int16','EdgePolarity','int16','ConversionTriggerSource','int16','ConversionEdgePolarity','int16','ConversionPeriod','double','BurstTriggerSource','int16','BurstEdgePolarity','int16','BurstSize','int16','DataSetOffset','int16','DataSetLength','int16','ReadMode','int16','SampleTime','double','StatusPortEnable','int16','TLCFileName','char','VoltageRange','int16')  RTIBlockParaDefault=struct('ADCSWStartDisable',0,'ModuleNo',1,'ChannelNo',1,'ConversionMode',1,'SampleMode',1,'TriggerSource',1,'EdgePolarity',1,'ConversionTriggerSource',2,'ConversionEdgePolarity',1,'ConversionPeriod',1e-6,'ConversionPeriodCheck',0,'BurstTriggerSource',1,'BurstEdgePolarity',1,'BurstSize',10,'BurstSizeCheck',0,'DataSetOffset',0,'DataSetOffsetCheck',0,'DataSetLength',1,'DataSetLengthCheck',0,'ReadMode',1,'SampleTime',-1,'SampleTimeCheck',1,'StatusPortEnable',0,'TLCFileName','rti1401adc_t4_adc','VoltageRange',1)
  ADC_TYPE4_BL6 : rti1401lib_adc_type4/ADC_TYPE4_BL1  DSProperties=struct('RTI',struct('Version',uint32(2),'BlockType',struct('isSLSource',uint8(1),'isSLSink',uint8(1),'isHWSource',uint8(0),'isHWSink',uint8(1),'isSetup',uint8(0),'isInline',uint8(1),'isNonInline',uint8(0),'isInterrupt',uint8(0),'isChannelwise',uint8(1)),'IOBoardType',{{'DS1401','STD','ADCT4'}},'UnitType','ADC','Identifier','ADC','DialogType','ML','BlockSet','NONE','SlaveProcessor','NONE'))  RTIBlockInterface=struct('InputPortsActive',0,'InputPortsWidth',int32(1),'InputPortsDataType',{{'SS_BOOLEAN'}},'InputPortsName',{{'Continue'}},'OutputPortsActive',[1 0],'OutputPortsWidth',int32([1 1]),'OutputPortsDataType',{{'SS_DOUBLE','SS_UINT8'}},'OutputPortsName',{{'ADC','Status'}},'DialogFcn','rti1401stdadct4adcgui','SampleTime',{{0.1}},'InitLevel',3,'IconTransparency','on','BlockDisplay',{{['ADC TP4\nModule: 1\nChannel: 6'],'center'}},'BlockName',struct('Token',{{'ADC_TYPE4_BL1'}}))  RTIBlockParameters=struct('ADCSWStartDisable',{{0,'OFF',[0 1]}},'ModuleNo',{{1,'OFF',[1 16]}},'ChannelNo',{{6,'OFF',[1 16]}},'ConversionMode',{{1,'OFF',[1 2]}},'SampleMode',{{1,'OFF',[1 2]}},'TriggerSource',{{1,'OFF',[1 5]}},'EdgePolarity',{{1,'OFF',[1 2]}},'ConversionTriggerSource',{{2,'OFF',[1 6]}},'ConversionEdgePolarity',{{1,'OFF',[1 2]}},'ConversionPeriod',{{'1e-06','OFF',[]}},'ConversionPeriodCheck',{{0,'OFF',[]}},'BurstTriggerSource',{{1,'OFF',[1 6]}},'BurstEdgePolarity',{{1,'OFF',[1 2]}},'BurstSize',{{'10','OFF',[]}},'BurstSizeCheck',{{0,'OFF',[]}},'DataSetOffset',{{'0','OFF',[]}},'DataSetOffsetCheck',{{0,'OFF',[]}},'DataSetLength',{{'1','OFF',[]}},'DataSetLengthCheck',{{0,'OFF',[]}},'ReadMode',{{1,'OFF',[1 2]}},'SampleTime',{{'100e-3','OFF',[-1 inf]}},'SampleTimeCheck',{{1,'OFF',[]}},'StatusPortEnable',{{0,'OFF',[0 1]}},'TLCFileName',{{'rti1401adc_t4_adc','OFF',[]}},'VoltageRange',{{1,'OFF',[1 2]}})  RTISFcnParameters=struct('ADCSWStartDisable','int32','ModuleNo','int32','ChannelNo','int16','ConversionMode','int16','SampleMode','int16','TriggerSource','int16','EdgePolarity','int16','ConversionTriggerSource','int16','ConversionEdgePolarity','int16','ConversionPeriod','double','BurstTriggerSource','int16','BurstEdgePolarity','int16','BurstSize','int16','DataSetOffset','int16','DataSetLength','int16','ReadMode','int16','SampleTime','double','StatusPortEnable','int16','TLCFileName','char','VoltageRange','int16')  RTIBlockParaDefault=struct('ADCSWStartDisable',0,'ModuleNo',1,'ChannelNo',1,'ConversionMode',1,'SampleMode',1,'TriggerSource',1,'EdgePolarity',1,'ConversionTriggerSource',2,'ConversionEdgePolarity',1,'ConversionPeriod',1e-6,'ConversionPeriodCheck',0,'BurstTriggerSource',1,'BurstEdgePolarity',1,'BurstSize',10,'BurstSizeCheck',0,'DataSetOffset',0,'DataSetOffsetCheck',0,'DataSetLength',1,'DataSetLengthCheck',0,'ReadMode',1,'SampleTime',-1,'SampleTimeCheck',1,'StatusPortEnable',0,'TLCFileName','rti1401adc_t4_adc','VoltageRange',1)
  ADC_TYPE4_BL7 : rti1401lib_adc_type4/ADC_TYPE4_BL1  DSProperties=struct('RTI',struct('Version',uint32(2),'BlockType',struct('isSLSource',uint8(1),'isSLSink',uint8(1),'isHWSource',uint8(0),'isHWSink',uint8(1),'isSetup',uint8(0),'isInline',uint8(1),'isNonInline',uint8(0),'isInterrupt',uint8(0),'isChannelwise',uint8(1)),'IOBoardType',{{'DS1401','STD','ADCT4'}},'UnitType','ADC','Identifier','ADC','DialogType','ML','BlockSet','NONE','SlaveProcessor','NONE'))  RTIBlockInterface=struct('InputPortsActive',0,'InputPortsWidth',int32(1),'InputPortsDataType',{{'SS_BOOLEAN'}},'InputPortsName',{{'Continue'}},'OutputPortsActive',[1 0],'OutputPortsWidth',int32([1 1]),'OutputPortsDataType',{{'SS_DOUBLE','SS_UINT8'}},'OutputPortsName',{{'ADC','Status'}},'DialogFcn','rti1401stdadct4adcgui','SampleTime',{{0.1}},'InitLevel',3,'IconTransparency','on','BlockDisplay',{{['ADC TP4\nModule: 1\nChannel: 7'],'center'}},'BlockName',struct('Token',{{'ADC_TYPE4_BL1'}}))  RTIBlockParameters=struct('ADCSWStartDisable',{{0,'OFF',[0 1]}},'ModuleNo',{{1,'OFF',[1 16]}},'ChannelNo',{{7,'OFF',[1 16]}},'ConversionMode',{{1,'OFF',[1 2]}},'SampleMode',{{1,'OFF',[1 2]}},'TriggerSource',{{1,'OFF',[1 5]}},'EdgePolarity',{{1,'OFF',[1 2]}},'ConversionTriggerSource',{{2,'OFF',[1 6]}},'ConversionEdgePolarity',{{1,'OFF',[1 2]}},'ConversionPeriod',{{'1e-06','OFF',[]}},'ConversionPeriodCheck',{{0,'OFF',[]}},'BurstTriggerSource',{{1,'OFF',[1 6]}},'BurstEdgePolarity',{{1,'OFF',[1 2]}},'BurstSize',{{'10','OFF',[]}},'BurstSizeCheck',{{0,'OFF',[]}},'DataSetOffset',{{'0','OFF',[]}},'DataSetOffsetCheck',{{0,'OFF',[]}},'DataSetLength',{{'1','OFF',[]}},'DataSetLengthCheck',{{0,'OFF',[]}},'ReadMode',{{1,'OFF',[1 2]}},'SampleTime',{{'100e-3','OFF',[-1 inf]}},'SampleTimeCheck',{{1,'OFF',[]}},'StatusPortEnable',{{0,'OFF',[0 1]}},'TLCFileName',{{'rti1401adc_t4_adc','OFF',[]}},'VoltageRange',{{1,'OFF',[1 2]}})  RTISFcnParameters=struct('ADCSWStartDisable','int32','ModuleNo','int32','ChannelNo','int16','ConversionMode','int16','SampleMode','int16','TriggerSource','int16','EdgePolarity','int16','ConversionTriggerSource','int16','ConversionEdgePolarity','int16','ConversionPeriod','double','BurstTriggerSource','int16','BurstEdgePolarity','int16','BurstSize','int16','DataSetOffset','int16','DataSetLength','int16','ReadMode','int16','SampleTime','double','StatusPortEnable','int16','TLCFileName','char','VoltageRange','int16')  RTIBlockParaDefault=struct('ADCSWStartDisable',0,'ModuleNo',1,'ChannelNo',1,'ConversionMode',1,'SampleMode',1,'TriggerSource',1,'EdgePolarity',1,'ConversionTriggerSource',2,'ConversionEdgePolarity',1,'ConversionPeriod',1e-6,'ConversionPeriodCheck',0,'BurstTriggerSource',1,'BurstEdgePolarity',1,'BurstSize',10,'BurstSizeCheck',0,'DataSetOffset',0,'DataSetOffsetCheck',0,'DataSetLength',1,'DataSetLengthCheck',0,'ReadMode',1,'SampleTime',-1,'SampleTimeCheck',1,'StatusPortEnable',0,'TLCFileName','rti1401adc_t4_adc','VoltageRange',1)
  ADC_TYPE4_BL8 : rti1401lib_adc_type4/ADC_TYPE4_BL1  DSProperties=struct('RTI',struct('Version',uint32(2),'BlockType',struct('isSLSource',uint8(1),'isSLSink',uint8(1),'isHWSource',uint8(0),'isHWSink',uint8(1),'isSetup',uint8(0),'isInline',uint8(1),'isNonInline',uint8(0),'isInterrupt',uint8(0),'isChannelwise',uint8(1)),'IOBoardType',{{'DS1401','STD','ADCT4'}},'UnitType','ADC','Identifier','ADC','DialogType','ML','BlockSet','NONE','SlaveProcessor','NONE'))  RTIBlockInterface=struct('InputPortsActive',0,'InputPortsWidth',int32(1),'InputPortsDataType',{{'SS_BOOLEAN'}},'InputPortsName',{{'Continue'}},'OutputPortsActive',[1 0],'OutputPortsWidth',int32([1 1]),'OutputPortsDataType',{{'SS_DOUBLE','SS_UINT8'}},'OutputPortsName',{{'ADC','Status'}},'DialogFcn','rti1401stdadct4adcgui','SampleTime',{{0.1}},'InitLevel',3,'IconTransparency','on','BlockDisplay',{{['ADC TP4\nModule: 1\nChannel: 8'],'center'}},'BlockName',struct('Token',{{'ADC_TYPE4_BL1'}}))  RTIBlockParameters=struct('ADCSWStartDisable',{{0,'OFF',[0 1]}},'ModuleNo',{{1,'OFF',[1 16]}},'ChannelNo',{{8,'OFF',[1 16]}},'ConversionMode',{{1,'OFF',[1 2]}},'SampleMode',{{1,'OFF',[1 2]}},'TriggerSource',{{1,'OFF',[1 5]}},'EdgePolarity',{{1,'OFF',[1 2]}},'ConversionTriggerSource',{{2,'OFF',[1 6]}},'ConversionEdgePolarity',{{1,'OFF',[1 2]}},'ConversionPeriod',{{'1e-06','OFF',[]}},'ConversionPeriodCheck',{{0,'OFF',[]}},'BurstTriggerSource',{{1,'OFF',[1 6]}},'BurstEdgePolarity',{{1,'OFF',[1 2]}},'BurstSize',{{'10','OFF',[]}},'BurstSizeCheck',{{0,'OFF',[]}},'DataSetOffset',{{'0','OFF',[]}},'DataSetOffsetCheck',{{0,'OFF',[]}},'DataSetLength',{{'1','OFF',[]}},'DataSetLengthCheck',{{0,'OFF',[]}},'ReadMode',{{1,'OFF',[1 2]}},'SampleTime',{{'100e-3','OFF',[-1 inf]}},'SampleTimeCheck',{{1,'OFF',[]}},'StatusPortEnable',{{0,'OFF',[0 1]}},'TLCFileName',{{'rti1401adc_t4_adc','OFF',[]}},'VoltageRange',{{1,'OFF',[1 2]}})  RTISFcnParameters=struct('ADCSWStartDisable','int32','ModuleNo','int32','ChannelNo','int16','ConversionMode','int16','SampleMode','int16','TriggerSource','int16','EdgePolarity','int16','ConversionTriggerSource','int16','ConversionEdgePolarity','int16','ConversionPeriod','double','BurstTriggerSource','int16','BurstEdgePolarity','int16','BurstSize','int16','DataSetOffset','int16','DataSetLength','int16','ReadMode','int16','SampleTime','double','StatusPortEnable','int16','TLCFileName','char','VoltageRange','int16')  RTIBlockParaDefault=struct('ADCSWStartDisable',0,'ModuleNo',1,'ChannelNo',1,'ConversionMode',1,'SampleMode',1,'TriggerSource',1,'EdgePolarity',1,'ConversionTriggerSource',2,'ConversionEdgePolarity',1,'ConversionPeriod',1e-6,'ConversionPeriodCheck',0,'BurstTriggerSource',1,'BurstEdgePolarity',1,'BurstSize',10,'BurstSizeCheck',0,'DataSetOffset',0,'DataSetOffsetCheck',0,'DataSetLength',1,'DataSetLengthCheck',0,'ReadMode',1,'SampleTime',-1,'SampleTimeCheck',1,'StatusPortEnable',0,'TLCFileName','rti1401adc_t4_adc','VoltageRange',1)
  Bus Creator : BusCreator  Inputs=8
  FlightRecorder1 : Subsystem
  FlightRecorder4 : Subsystem
  Gain : Gain
  Spannungsteiler : Gain  Gain=5 * 5.512195 * 1.06451
  Terminator : Terminator
  Umrechnung ADC-Widerstand : Subsystem
  Umrechnung ADC-Widerstand1 : Subsystem
  Umrechnung Widerstand - Temperatur NTC : Subsystem
  Umrechnung Widerstand - Temperatur NTC1 : Subsystem
  AI : Outport
  wires:
  ADC_TYPE4_BL1/1 -> Bus Creator/1  "Ch1"
  ADC_TYPE4_BL2/1 -> Bus Creator/2  "Ch2"
  ADC_TYPE4_BL3/1 -> Bus Creator/3  "Ch3"
  ADC_TYPE4_BL4/1 -> Bus Creator/4  "Ch4"
  ADC_TYPE4_BL5/1 -> Umrechnung ADC-Widerstand/1(ADC)  "Ch5_Wassertemp"
  ADC_TYPE4_BL6/1 -> Spannungsteiler/1  "Ch6"
  Bus Creator/1 -> Gain/1, AI/1  "AI"
  Gain/1 -> Terminator/1
  ADC_TYPE4_BL8/1 -> Bus Creator/8  "Ch8"
  Umrechnung ADC-Widerstand/1(R) -> Umrechnung Widerstand - Temperatur NTC/1(R)
  Umrechnung Widerstand - Temperatur NTC/1(Temperatur) -> FlightRecorder1/1(In1), Bus Creator/5  "Wassertemp"
  ADC_TYPE4_BL7/1 -> Umrechnung ADC-Widerstand1/1(ADC)  "Ch7_MOSFET_Temp"
  Spannungsteiler/1 -> FlightRecorder4/1(In1), Bus Creator/6, Umrechnung ADC-Widerstand1/2(Uref[V]), Umrechnung ADC-Widerstand/2(Uref[V])  "UBatt"
  Umrechnung ADC-Widerstand1/1(R) -> Umrechnung Widerstand - Temperatur NTC1/1(R)
  Umrechnung Widerstand - Temperatur NTC1/1(Temperatur) -> Bus Creator/7  "Mosfet Temp"
